simulink model "SCR_SiLS_R3"  (R2023a)
settings: Solver=VariableStepAuto  StartTime=0.0  StopTime=T_sim_end  RelTol=1e-3
model workspace (MAT data in the model file):
  ConnVar.ipAddress = '192.168.0.153'
  ConnVar.user = 'M1'
  ConnVar.pwd = [145 145 158 146 151 156 158 157]
  ConnVar.targetHandle = 0
values from neighbouring files (symbols this model uses):
  Ts_com = 0.1    [Script_individual_test_init.m]
undefined symbols (not defined in the file or in its folder): var01, var02, var03, var04, var05, var1, var2, var3, var4
libraries: M1SWBlocks x6, simulink x4
settings Model: Creator=CHSE  LastModifiedBy=gione
settings DebuggingCC: UnconnectedInputMsg=warning  UnconnectedOutputMsg=warning  UnconnectedLineMsg=warning
settings ModelReferenceCC: EnableRefExpFcnMdlSchedulingChecks=on
settings RTWCC: DLArmComputeVersion=19.05

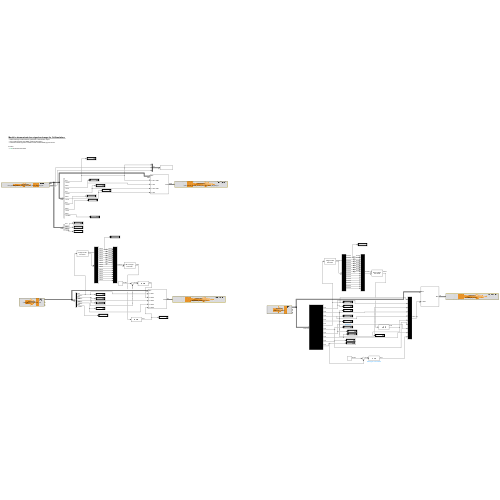
[thumbnail: Simulink's stored preview of the top-level diagram]
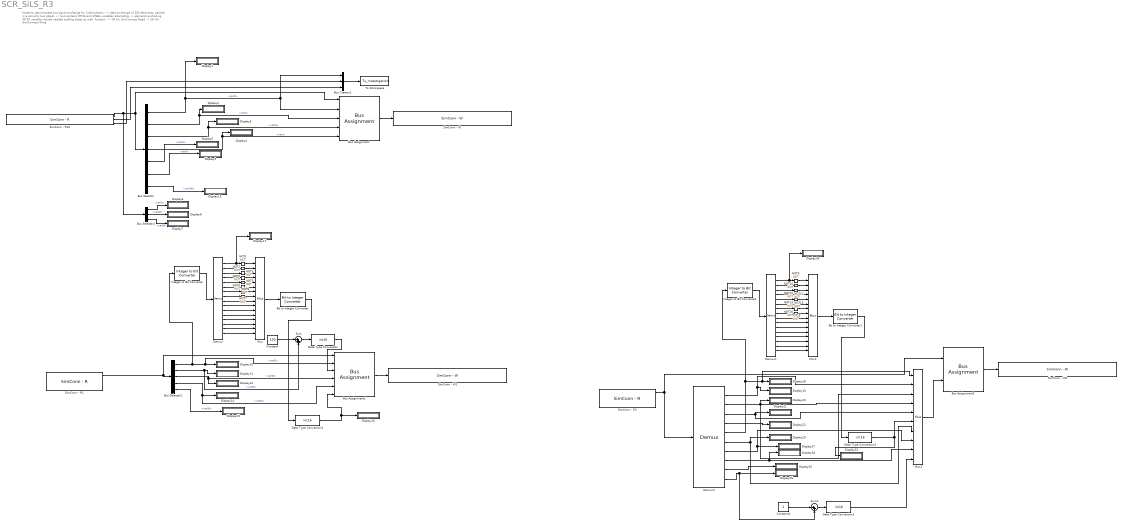
== system SCR_SiLS_R3 ==
  note: Model to demonstrate bus signal exchange for CoSimulation:
      | -> data exchange of 200 elements, packed in a simulink bus object.
      | -> bus contains INT16 and LREAL variables alternating
      | -> elements exchaning INT16 variable include needed stuffing bytes as well.
      |
      | function:
      | -> OK für SimConnect Read
      | -> OK für SimConnect Write
  Bit to Integer Converter : simulink/Logic and Bit Operations/Bit to Integer Converter  nbits=16  bitOrder=LSB first  signedOutputValues=Unsigned  outDtype=Inherit via internal rule  outDtypeSigned=Inherit via internal rule
  Bit to Integer Converter1 : simulink/Logic and Bit Operations/Bit to Integer Converter  nbits=16  bitOrder=LSB first  signedOutputValues=Unsigned  outDtype=Inherit via internal rule  outDtypeSigned=Inherit via internal rule
  Bus Assignment : BusAssignment  AssignedSignals=var1.var01,var2,var3.var01,var4
  Bus Assignment1 : BusAssignment  AssignedSignals=var01,var02,var03,var04,var05
  Bus Assignment2 : BusAssignment  AssignedSignals=data
  Bus Creator1 : BusCreator  Inputs=3
  Bus Selector : BusSelector  OutputSignals=var1.var01,var2,var3.var01,var4,var5.var01,var6,var200
  Bus Selector1 : BusSelector  OutputSignals=var1.var01,var1.var02,var1.var03
  Bus Selector2 : BusSelector  OutputSignals=var01,var02,var03,var04,var05
  Constant : Constant  Value=100
  Constant1 : Constant
  Data Type Conversion{,1..3} (4 alike) : DataTypeConversion  OutDataTypeStr=int16  SaturateOnIntegerOverflow=off  RndMeth=Floor
  Demux : Demux  Outputs=16
  Demux1 : Demux  Outputs=16
  Demux2 : Demux  Outputs=10
  Display{1..29} (29 alike) : Display
      Display12 settings: Format=decimal (Stored Integer)
      Display20 settings: Format=decimal (Stored Integer)
  Integer to Bit Converter : simulink/Logic and Bit Operations/Integer to Bit Converter  nbits=16  signedInputValues=Unsigned  bitOrder=LSB first  outDtype=boolean
  Integer to Bit Converter1 : simulink/Logic and Bit Operations/Integer to Bit Converter  nbits=16  signedInputValues=Unsigned  bitOrder=LSB first  outDtype=boolean
  Mux : Mux  Inputs=16
  Mux1 : Mux  Inputs=16
  Mux2 : Mux  Inputs=10
  NOT{1..16} (16 alike) : Logic  Operator=NOT  IconShape=distinctive  AllPortsSameDT=off  OutDataTypeStr=boolean
  SimConn - R1 : M1SWBlocks/SimConn Blocks/SimConn - R  connVarName=ConnVar  InswModuleName='NONOXR4'  swModuleName=NONOXR4  InvarName='.var2_INT16_scalar_bus_out'  varName=.var2_INT16_scalar_bus_out  varDataType=Bus: INT16_10Byte_aligned  enRetOutput=on  enGetTrigger=off  getTrigger=rising  valDurLostConn=Zero  internalVal=0  DataDim=1  enSampTimMon=on  sampleTime=Ts_com
      settings: SourceProductName=Bachmann M1 Software
  SimConn - R10 : M1SWBlocks/SimConn Blocks/SimConn - R  connVarName=ConnVar  InswModuleName='NONOXR4'  swModuleName=NONOXR4  InvarName='.var1_INT16_LREAL_scalar_bus_200_mixed_aligned_out'  varName=.var1_INT16_LREAL_scalar_bus_200_mixed_aligned_out  varDataType=Bus: Bus_exchange_INT16_LREAL_mixed_scalar_200_aligned  enRetOutput=on  enGetTrigger=off  getTrigger=rising  valDurLostConn=Zero  internalVal=0  DataDim=1  enSampTimMon=on  sampleTime=Ts_com
      settings: SourceProductName=Bachmann M1 Software
  SimConn - R2 : M1SWBlocks/SimConn Blocks/SimConn - R  connVarName=ConnVar  InswModuleName='NONOXR4'  swModuleName=NONOXR4  InvarName='.Sils_DO_Comm'  varName=.Sils_DO_Comm  varDataType=Bus: IOSim_typ  enRetOutput=on  enGetTrigger=off  getTrigger=rising  valDurLostConn=Zero  internalVal=0  DataDim=1  enSampTimMon=on  sampleTime=Ts_com
      settings: SourceProductName=Bachmann M1 Software
  SimConn - W : M1SWBlocks/SimConn Blocks/SimConn - W  connVarName=ConnVar  InswModuleName='NONOXR4'  swModuleName=NONOXR4  InvarName='.var1_INT16_LREAL_scalar_bus_200_mixed_aligned_in'  varName=.var1_INT16_LREAL_scalar_bus_200_mixed_aligned_in  varDataType=Bus: Bus_exchange_INT16_LREAL_mixed_scalar_200_aligned  enRetOutput=off  enGetTrigger=off  getTrigger=rising  enSampTimMon=off
      settings: SourceProductName=Bachmann M1 Software
  SimConn - W1 : M1SWBlocks/SimConn Blocks/SimConn - W  connVarName=ConnVar  InswModuleName='NONOXR4'  swModuleName=NONOXR4  InvarName='.var2_INT16_scalar_bus_in'  varName=.var2_INT16_scalar_bus_in  varDataType=Bus: INT16_10Byte_aligned  enRetOutput=off  enGetTrigger=off  getTrigger=rising  enSampTimMon=off
      settings: SourceProductName=Bachmann M1 Software
  SimConn - W2 : M1SWBlocks/SimConn Blocks/SimConn - W  connVarName=ConnVar  InswModuleName='NONOXR4'  swModuleName=NONOXR4  InvarName='.Sils_DI_Comm'  varName=.Sils_DI_Comm  varDataType=Bus: IOSim_typ  enRetOutput=off  enGetTrigger=off  getTrigger=rising  enSampTimMon=off
      settings: SourceProductName=Bachmann M1 Software
  Sum : Sum  Inputs=|++
  Sum1 : Sum  Inputs=|++
  To Workspace : ToWorkspace  VariableName=Ts_investigation  SaveFormat=Timeseries  SampleTime=Ts_com
  wires:
  Bus Selector/2 -> Display2/1, Bus Assignment/3  "<var2>"
  Bus Selector/3 -> Display3/1, Bus Assignment/4  "<var01>"
  Bus Selector/4 -> Display4/1, Bus Assignment/5  "<var4>"
  Bus Creator1/1 -> To Workspace/1
  Bus Selector/1 -> Display1/1, Bus Assignment/2, Bus Creator1/1  "<var01>"
  SimConn - R10/2 -> Bus Creator1/3
  SimConn - R10/1 -> Bus Selector1/1, Bus Selector/1, Bus Assignment/1
  Bus Selector1/1 -> Display6/1  "<var01>"
  Bus Selector1/3 -> Display7/1  "<var03>"
  Bus Selector1/2 -> Display8/1  "<var02>"
  Bus Selector/5 -> Display5/1  "<var01>"
  Bus Selector/6 -> Display9/1  "<var6>"
  Bus Selector/7 -> Display13/1  "<var200>"
  SimConn - R10/3 -> Bus Creator1/2
  Bus Assignment/1 -> SimConn - W/1
  Bus Selector2/2 -> Sum/2, Display11/1  "<var02>"
  Bus Selector2/3 -> Display12/1, Bus Assignment1/4  "<var03>"
  SimConn - R1/1 -> Bus Assignment1/1, Bus Selector2/1
  Bus Selector2/1 -> Integer to Bit Converter/1, Bus Assignment1/2, Display10/1  "<var01>"
  Bus Assignment1/1 -> SimConn - W1/1
  Bus Selector2/4 -> Bus Assignment1/5, Display14/1  "<var04>"
  Bus Selector2/5 -> Display15/1  "<var05>"
  Constant/1 -> Sum/1
  Data Type Conversion/1 -> Bus Assignment1/3
  Sum/1 -> Data Type Conversion/1
  Data Type Conversion1/1 -> Display16/1, Bus Assignment1/6
  Bit to Integer Converter/1 -> Data Type Conversion1/1
  Integer to Bit Converter/1 -> Demux/1
  Demux/1 -> Display17/1, NOT1/1
  Demux/2 -> NOT2/1
  Demux/4 -> NOT4/1
  Demux/3 -> NOT3/1
  Demux/6 -> NOT6/1
  Demux/5 -> NOT5/1
  Demux/8 -> NOT8/1
  Demux/7 -> NOT7/1
  Demux/10 -> Mux/10
  Demux/11 -> Mux/11
  Demux/12 -> Mux/12
  Demux/9 -> Mux/9
  Demux/13 -> Mux/13
  Demux/14 -> Mux/14
  Demux/15 -> Mux/15
  Demux/16 -> Mux/16
  NOT8/1 -> Mux/8
  NOT7/1 -> Mux/7
  NOT6/1 -> Mux/6
  NOT5/1 -> Mux/5
  NOT4/1 -> Mux/4
  NOT3/1 -> Mux/3
  NOT2/1 -> Mux/2
  NOT1/1 -> Mux/1
  Mux/1 -> Bit to Integer Converter/1
  Demux1/7 -> NOT15/1
  Demux1/2 -> NOT10/1
  NOT16/1 -> Mux1/8
  Demux1/6 -> NOT14/1
  Demux1/12 -> Mux1/12
  NOT10/1 -> Mux1/2
  Demux1/13 -> Mux1/13
  NOT13/1 -> Mux1/5
  Demux1/9 -> Mux1/9
  Integer to Bit Converter1/1 -> Demux1/1
  Demux1/14 -> Mux1/14
  NOT9/1 -> Mux1/1
  Mux1/1 -> Bit to Integer Converter1/1
  Bit to Integer Converter1/1 -> Data Type Conversion3/1
  Demux1/4 -> NOT12/1
  Demux1/16 -> Mux1/16
  Demux2/5 -> Integer to Bit Converter1/1, Mux2/1, Display18/1
  Demux1/11 -> Mux1/11
  Demux1/10 -> Mux1/10
  NOT14/1 -> Mux1/6
  Demux2/3 -> Mux2/5, Display21/1
  Data Type Conversion3/1 -> Mux2/6, Display23/1
  NOT12/1 -> Mux1/4
  Demux1/3 -> NOT11/1
  Constant1/1 -> Sum1/1
  Demux2/4 -> Display22/1
  Demux1/1 -> Display24/1, NOT9/1
  Sum1/1 -> Data Type Conversion2/1
  Demux2/2 -> Display20/1, Mux2/3, Mux2/4
  Demux2/1 -> Mux2/2, Display19/1
  NOT11/1 -> Mux1/3
  Demux1/5 -> NOT13/1
  NOT15/1 -> Mux1/7
  Demux1/15 -> Mux1/15
  Demux1/8 -> NOT16/1
  SimConn - R2/1 -> Bus Assignment2/1, Demux2/1
  Demux2/9 -> Display25/1
  Demux2/10 -> Sum1/2, Display26/1
  Demux2/8 -> Mux2/9, Display28/1
  Demux2/7 -> Mux2/8, Display27/1
  Demux2/6 -> Mux2/7, Display29/1
  Mux2/1 -> Bus Assignment2/2
  Bus Assignment2/1 -> SimConn - W2/1
  Data Type Conversion2/1 -> Mux2/10
